simulink model "parte1_eje12_controlP_v2013a"  (Simulink 8.1)
settings: Solver=ode45  SolverMode=SingleTasking  StartTime=0.0  StopTime=10.0  RelTol=1e-3
libraries: simulink x1
settings Model: Creator=cjuar  LastModifiedBy=cjuar  CovMetricSettings=dwe  CovHtmlReporting=off  covSaveCumulativeToWorkspaceVar=off  CovSaveSingleToWorkspaceVar=off  CovExternalEMLEnable=on
settings DataIOCC: LimitDataPoints=off  SaveFormat=StructureWithTime  SignalLoggingSaveFormat=Dataset
settings OptimizationCC: ExpressionDepthLimit=128
settings DebuggingCC: UnderspecifiedInitializationDetection=Simplified  MergeDetectMultiDrivingBlocksExec=error  SolverPrmCheckMsg=none  FcnCallInpInsideContextMsg=EnableAllAsError  FrameProcessingCompatibilityMsg=error  StateNameClashWarn=none  SFUnexpectedBacktrackingDiag=error  SFNoUnconditionalDefaultTransitionDiag=error
settings HardwareCC: ProdBitPerPointer=64  ProdLargestAtomicFloat=Float  ProdIntDivRoundTo=Zero  ProdEndianess=LittleEndian  ProdHWDeviceType=Specified
settings ModelReferenceCC: PropagateSignalLabelsOutOfModel=on
settings GRTTargetCC: CodeReplacementLibrary=C99 (ISO)  GeneratePreprocessorConditionals=Use local settings  CombineOutputUpdateFcns=on  GRTInterface=off

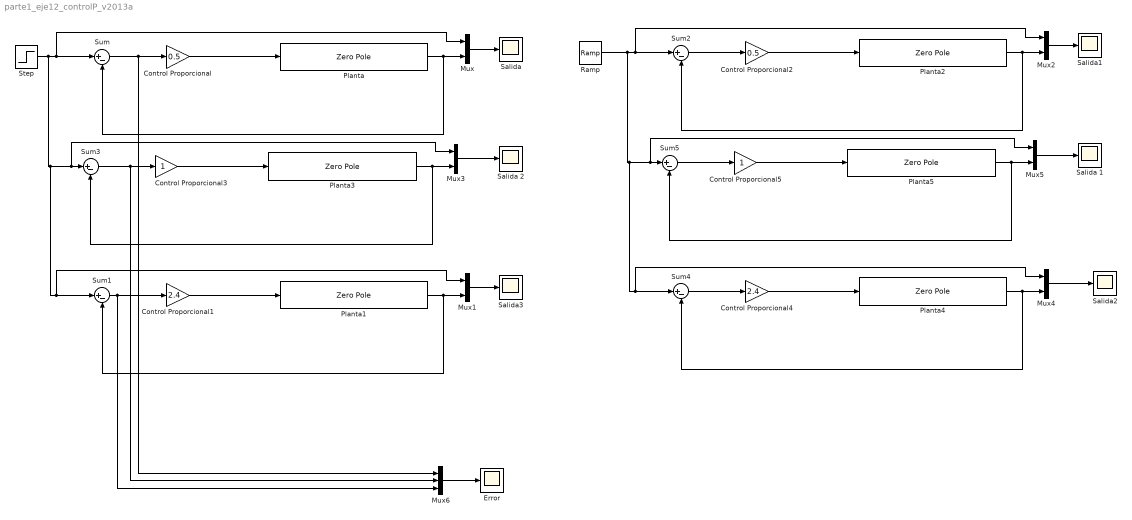
== system parte1_eje12_controlP_v2013a ==
  Control Proporcional : Gain  Gain=0.5
  Control Proporcional1 : Gain  Gain=2.4
  Control Proporcional2 : Gain  Gain=0.5
  Control Proporcional3 : Gain
  Control Proporcional4 : Gain  Gain=2.4
  Control Proporcional5 : Gain
  Error : Scope
      settings: TimeRange=auto  ShowLegends=on  MaxDataPoints=5000  SaveToWorkspace=off  SaveName=ScopeData6  YMin=-1.1551  YMax=1.23946  SampleTime=-1
  Mux{,1..5} (6 alike) : Mux  Inputs=2
  Mux6 : Mux  Inputs=3
  Planta{,1..5} (6 alike) : ZeroPole  Zeros=[]  Poles=[0 -6 -18]  Gain=1080
  Ramp : simulink/Sources/Ramp  slope=1  start=0  X0=0
  Salida{,1..3} (4 alike) : Scope
      Salida settings: TimeRange=auto  ShowLegends=on  MaxDataPoints=5000  SaveToWorkspace=off  SaveName=ScopeData  YMin=-0.15682  YMax=1.41134  SampleTime=-1
      Salida1 settings: TimeRange=auto  ShowLegends=on  MaxDataPoints=5000  SaveToWorkspace=off  SaveName=ScopeData4  YMin=-1.25  YMax=11.25  SampleTime=-1
      Salida2 settings: TimeRange=auto  ShowLegends=on  MaxDataPoints=5000  SaveToWorkspace=off  SaveName=ScopeData5  YMin=-1.25  YMax=11.25  SampleTime=-1
      Salida3 settings: TimeRange=auto  ShowLegends=on  MaxDataPoints=5000  SaveToWorkspace=off  YMin=-0.23946  YMax=2.1551  SampleTime=-1
  Salida 1 : Scope
      settings: TimeRange=auto  ShowLegends=on  MaxDataPoints=5000  SaveToWorkspace=off  SaveName=ScopeData2  YMin=-1.25  YMax=11.25  SampleTime=-1
  Salida 2 : Scope
      settings: TimeRange=auto  ShowLegends=on  MaxDataPoints=5000  SaveToWorkspace=off  SaveName=ScopeData3  YMin=-0.18802  YMax=1.69214  SampleTime=-1
  Step : Step  SampleTime=0
  Sum{,1..5} (6 alike) : Sum  Inputs=|+-
  wires:
  Control Proporcional/1 -> Planta/1
  Sum/1 -> Control Proporcional/1, Mux6/1
  Planta/1 -> Sum/2, Mux/2
  Mux/1 -> Salida/1
  Mux1/1 -> Salida3/1
  Planta1/1 -> Mux1/2, Sum1/2
  Sum1/1 -> Mux6/3, Control Proporcional1/1
  Control Proporcional1/1 -> Planta1/1
  Step/1 -> Mux3/1, Sum3/1, Sum1/1, Mux1/1, Mux/1, Sum/1
  Mux3/1 -> Salida 2/1
  Planta3/1 -> Mux3/2, Sum3/2
  Sum3/1 -> Mux6/2, Control Proporcional3/1
  Control Proporcional3/1 -> Planta3/1
  Sum2/1 -> Control Proporcional2/1
  Control Proporcional2/1 -> Planta2/1
  Planta2/1 -> Sum2/2, Mux2/2
  Ramp/1 -> Mux5/1, Sum5/1, Sum4/1, Mux4/1, Mux2/1, Sum2/1
  Sum5/1 -> Control Proporcional5/1
  Control Proporcional5/1 -> Planta5/1
  Planta5/1 -> Mux5/2, Sum5/2
  Mux5/1 -> Salida 1/1
  Control Proporcional4/1 -> Planta4/1
  Sum4/1 -> Control Proporcional4/1
  Mux2/1 -> Salida1/1
  Mux4/1 -> Salida2/1
  Planta4/1 -> Mux4/2, Sum4/2
  Mux6/1 -> Error/1
